simulink library "aec"  (Simulink 8.1)
settings: Solver=ode45  StartTime=0.0  StopTime=10.0  RelTol=1e-3
undefined symbols (not defined in the file or in its folder): ENUM_KEYSWITCH_ON, ENUM_SENSORSTATE_NORMAL, FALSE
settings Model: Creator=xsellart  LastModifiedBy=AT015555

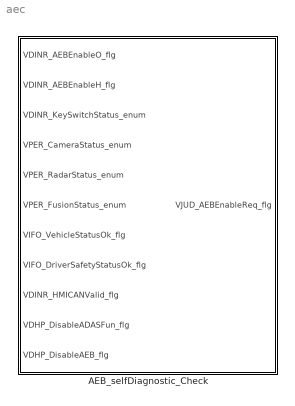
== system aec ==
  AEB_selfDiagnostic_Check : Subsystem

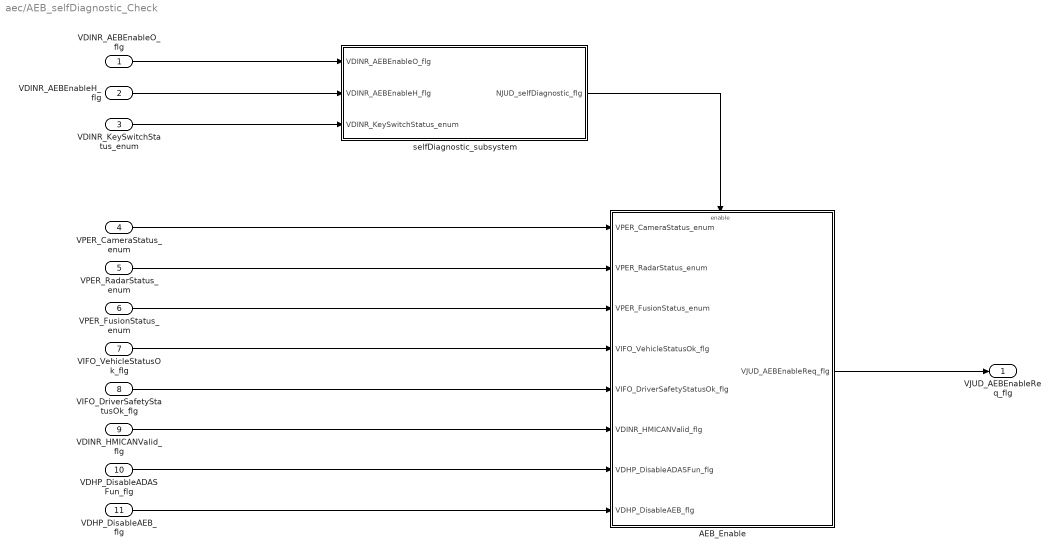
== system aec/AEB_selfDiagnostic_Check ==
  VDINR_AEBEnableO_flg : Inport
  VDINR_AEBEnableH_flg : Inport  Port=2
  VDINR_KeySwitchStatus_enum : Inport  Port=3
  VPER_CameraStatus_enum : Inport  Port=4
  VPER_RadarStatus_enum : Inport  Port=5
  VPER_FusionStatus_enum : Inport  Port=6
  VIFO_VehicleStatusOk_flg : Inport  Port=7
  VIFO_DriverSafetyStatusOk_flg : Inport  Port=8
  VDINR_HMICANValid_flg : Inport  Port=9
  VDHP_DisableADASFun_flg : Inport  Port=10
  VDHP_DisableAEB_flg : Inport  Port=11
  AEB_Enable : Subsystem
  selfDiagnostic_subsystem : Subsystem
  VJUD_AEBEnableReq_flg : Outport
  wires:
  AEB_Enable/1(VJUD_AEBEnableReq_flg) -> VJUD_AEBEnableReq_flg/1
  VIFO_DriverSafetyStatusOk_flg/1 -> AEB_Enable/5(VIFO_DriverSafetyStatusOk_flg)
  VDINR_HMICANValid_flg/1 -> AEB_Enable/6(VDINR_HMICANValid_flg)
  VIFO_VehicleStatusOk_flg/1 -> AEB_Enable/4(VIFO_VehicleStatusOk_flg)
  VPER_FusionStatus_enum/1 -> AEB_Enable/3(VPER_FusionStatus_enum)
  VPER_RadarStatus_enum/1 -> AEB_Enable/2(VPER_RadarStatus_enum)
  VPER_CameraStatus_enum/1 -> AEB_Enable/1(VPER_CameraStatus_enum)
  selfDiagnostic_subsystem/1(NJUD_selfDiagnostic_flg) -> AEB_Enable/Enable
  VDHP_DisableADASFun_flg/1 -> AEB_Enable/7(VDHP_DisableADASFun_flg)
  VDHP_DisableAEB_flg/1 -> AEB_Enable/8(VDHP_DisableAEB_flg)
  VDINR_AEBEnableO_flg/1 -> selfDiagnostic_subsystem/1(VDINR_AEBEnableO_flg)
  VDINR_AEBEnableH_flg/1 -> selfDiagnostic_subsystem/2(VDINR_AEBEnableH_flg)
  VDINR_KeySwitchStatus_enum/1 -> selfDiagnostic_subsystem/3(VDINR_KeySwitchStatus_enum)

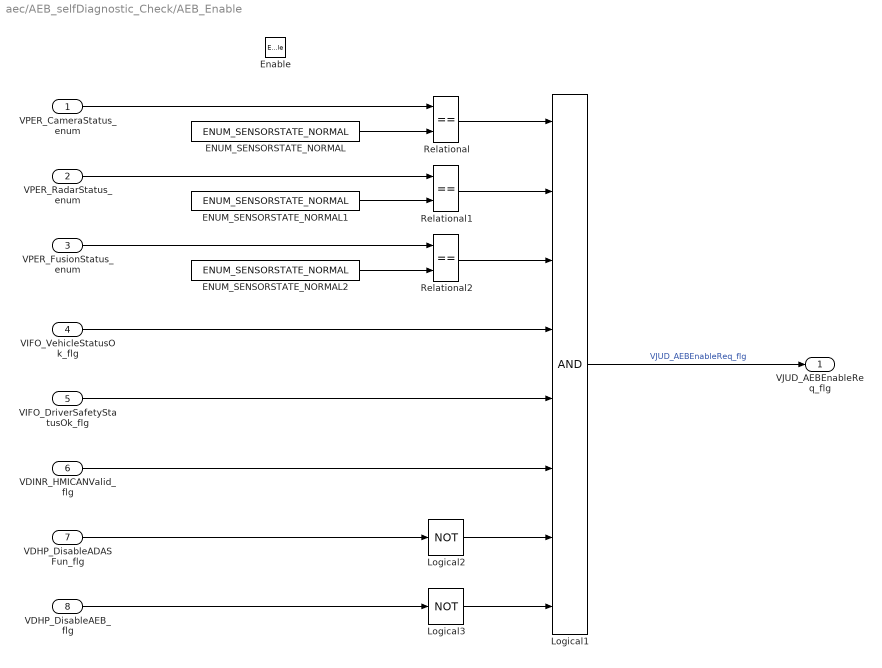
== system aec/AEB_selfDiagnostic_Check/AEB_Enable ==
  VPER_CameraStatus_enum : Inport
  VPER_RadarStatus_enum : Inport  Port=2
  VPER_FusionStatus_enum : Inport  Port=3
  VIFO_VehicleStatusOk_flg : Inport  Port=4
  VIFO_DriverSafetyStatusOk_flg : Inport  Port=5
  VDINR_HMICANValid_flg : Inport  Port=6
  VDHP_DisableADASFun_flg : Inport  Port=7
  VDHP_DisableAEB_flg : Inport  Port=8
  Enable : EnablePort
  ENUM_SENSORSTATE_NORMAL : Constant  Value=ENUM_SENSORSTATE_NORMAL  OutDataTypeStr=uint8
  ENUM_SENSORSTATE_NORMAL1 : Constant  Value=ENUM_SENSORSTATE_NORMAL  OutDataTypeStr=uint8
  ENUM_SENSORSTATE_NORMAL2 : Constant  Value=ENUM_SENSORSTATE_NORMAL  OutDataTypeStr=uint8
  Logical1 : Logic  Inputs=8  AllPortsSameDT=off  OutDataTypeStr=boolean
  Logical2 : Logic  Operator=NOT  Inputs=6  AllPortsSameDT=off  OutDataTypeStr=boolean
  Logical3 : Logic  Operator=NOT  Inputs=6  AllPortsSameDT=off  OutDataTypeStr=boolean
  Relational : RelationalOperator  Operator===  OutDataTypeStr=boolean
  Relational1 : RelationalOperator  Operator===  OutDataTypeStr=boolean
  Relational2 : RelationalOperator  Operator===  OutDataTypeStr=boolean
  VJUD_AEBEnableReq_flg : Outport  OutputWhenDisabled=reset  InitialOutput=FALSE
  wires:
  Logical1/1 -> VJUD_AEBEnableReq_flg/1  "VJUD_AEBEnableReq_flg"
  Relational2/1 -> Logical1/3
  Relational1/1 -> Logical1/2
  Relational/1 -> Logical1/1
  VIFO_VehicleStatusOk_flg/1 -> Logical1/4
  ENUM_SENSORSTATE_NORMAL2/1 -> Relational2/2
  VPER_FusionStatus_enum/1 -> Relational2/1
  ENUM_SENSORSTATE_NORMAL1/1 -> Relational1/2
  VPER_RadarStatus_enum/1 -> Relational1/1
  ENUM_SENSORSTATE_NORMAL/1 -> Relational/2
  VPER_CameraStatus_enum/1 -> Relational/1
  VIFO_DriverSafetyStatusOk_flg/1 -> Logical1/5
  VDINR_HMICANValid_flg/1 -> Logical1/6
  VDHP_DisableADASFun_flg/1 -> Logical2/1
  VDHP_DisableAEB_flg/1 -> Logical3/1
  Logical2/1 -> Logical1/7
  Logical3/1 -> Logical1/8

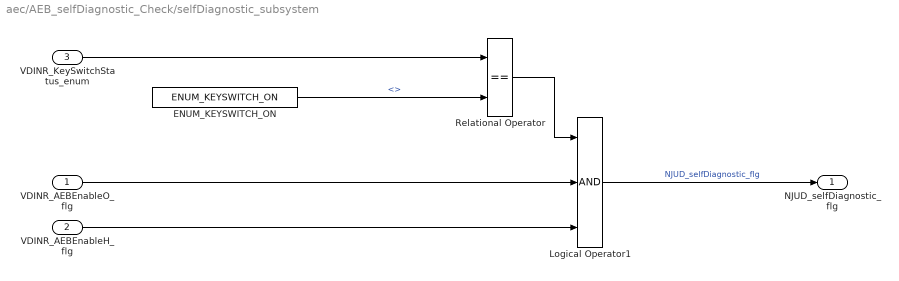
== system aec/AEB_selfDiagnostic_Check/selfDiagnostic_subsystem ==
  VDINR_AEBEnableO_flg : Inport
  VDINR_AEBEnableH_flg : Inport  Port=2
  VDINR_KeySwitchStatus_enum : Inport  Port=3
  ENUM_KEYSWITCH_ON : Constant  Value=ENUM_KEYSWITCH_ON  OutDataTypeStr=uint8
  Logical Operator1 : Logic  Inputs=3  AllPortsSameDT=off  OutDataTypeStr=boolean
  Relational Operator : RelationalOperator  Operator===  OutDataTypeStr=boolean
  NJUD_selfDiagnostic_flg : Outport
  wires:
  VDINR_KeySwitchStatus_enum/1 -> Relational Operator/1
  ENUM_KEYSWITCH_ON/1 -> Relational Operator/2  "<>"
  Relational Operator/1 -> Logical Operator1/1
  VDINR_AEBEnableH_flg/1 -> Logical Operator1/3
  VDINR_AEBEnableO_flg/1 -> Logical Operator1/2
  Logical Operator1/1 -> NJUD_selfDiagnostic_flg/1  "NJUD_selfDiagnostic_flg"
